simulink model "Type2FuzzyLogicSystems"  (R2012b)
settings: Solver=FixedStepDiscrete  StartTime=0.0  StopTime=10.0  FixedStep=0.1  RelTol=1e-3
libraries: Fuzzy_Type2_Lib x1
settings Model: Creator=u11f99  LastModifiedBy=u11f99

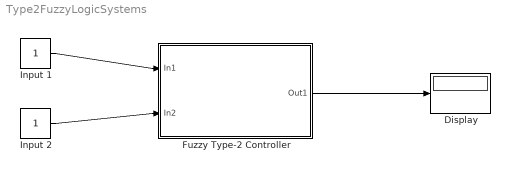
== system Type2FuzzyLogicSystems ==
  Display : Display
  Fuzzy Type-2 Controller : Subsystem
  Input 1 : Constant  SampleTime=-1
  Input 2 : Constant  SampleTime=-1
  wires:
  Input 1/1 -> Fuzzy Type-2 Controller/1(In1)
  Input 2/1 -> Fuzzy Type-2 Controller/2(In2)
  Fuzzy Type-2 Controller/1(Out1) -> Display/1

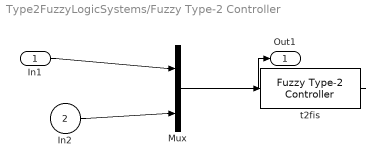
== system Type2FuzzyLogicSystems/Fuzzy Type-2 Controller ==
  In1 : Inport
  In2 : Inport  Port=2  SampleTime=0
  Mux : Mux  Inputs=2
  t2fis : Fuzzy_Type2_Lib/Fuzzy Type-2 Controller  t2fisSim=t2fisSim
  Out1 : Outport
  wires:
  In1/1 -> Mux/1
  In2/1 -> Mux/2
  Mux/1 -> t2fis/1
  t2fis/1 -> Out1/1
